simulink model "DPA_6bitDAC_MIXER_INL"  (R2015b)
settings: Solver=FixedStepDiscrete  SolverMode=SingleTasking  StartTime=0.0  StopTime=1/fs*(4*nn+ni)  RelTol=1e-3  AbsTol=1e-6
values from neighbouring files (symbols this model uses):
  AM = 1    [load_6bit_DPA_Mixerpsd_INL.m]
  Fc = 6.5e9    (= 6500000000)    [load_6bit_DPA_Mixerpsd_INL.m]
  fin1 = fs/nn*floor(fin1/fs*nn)    [load_6bit_DPA_Mixerpsd_INL.m]
  fin2 = fs/nn*floor(fin2/fs*nn)    [load_6bit_DPA_Mixerpsd_INL.m]
  fin3 = fs/nn*floor(fin3/fs*nn)    [load_6bit_DPA_Mixerpsd_INL.m]
  fin4 = fs/nn*floor(fin4/fs*nn)    [load_6bit_DPA_Mixerpsd_INL.m]
  fin5 = fs/nn*floor(fin5/fs*nn)    [load_6bit_DPA_Mixerpsd_INL.m]
  fin6 = fs/nn*floor(fin6/fs*nn)    [load_6bit_DPA_Mixerpsd_INL.m]
  fin7 = fs/nn*floor(fin7/fs*nn)    [load_6bit_DPA_Mixerpsd_INL.m]
  fin8 = fs/nn*floor(fin8/fs*nn)    [load_6bit_DPA_Mixerpsd_INL.m]
  fs = Fc*4    (= 26000000000)    [load_6bit_DPA_Mixerpsd_INL.m]
  g1 = (1-2^-32)/8    (= 0.124999999971)    [load_6bit_DPA_Mixerpsd_INL.m]
  NUM = [1,1]    [load_6bit_DPA_Mixerpsd_INL.m]
undefined symbols (not defined in the file or in its folder): RR6bit, RR6bit_ideal
settings Model: ExtModeTrigMode=oneshot  ExtModeArmWhenConnect=off  Creator=john  LastModifiedBy=John_dell_NB2019
settings DataIOCC: LimitDataPoints=off  SaveFormat=Array  SignalLoggingSaveFormat=ModelDataLogs
settings OptimizationCC: BlockReduction=off  BooleanDataType=off
settings DebuggingCC: SaveWithParameterizedLinksMsg=none  UnderspecifiedInitializationDetection=Classic  MergeDetectMultiDrivingBlocksExec=none  SignalResolutionControl=TryResolveAllWithWarning  MultiTaskDSMMsg=warning  MultiTaskCondExecSysMsg=none  StateNameClashWarn=warning
settings HardwareCC: ProdBitPerPointer=32  ProdLargestAtomicFloat=None  ProdIntDivRoundTo=Undefined  ProdEndianess=Unspecified  ProdWordSize=32  ProdHWDeviceType=32-bit Generic  TargetBitPerPointer=64  TargetLongLongMode=on  TargetIntDivRoundTo=Zero  TargetEndianess=LittleEndian  TargetWordSize=64  TargetHWDeviceType=MATLAB Host  ProdEqTarget=off
settings GRTTargetCC: GeneratePreprocessorConditionals=Disable all  CombineOutputUpdateFcns=off  GRTInterface=on
settings ConfigComp: CovModelRefEnable=Off

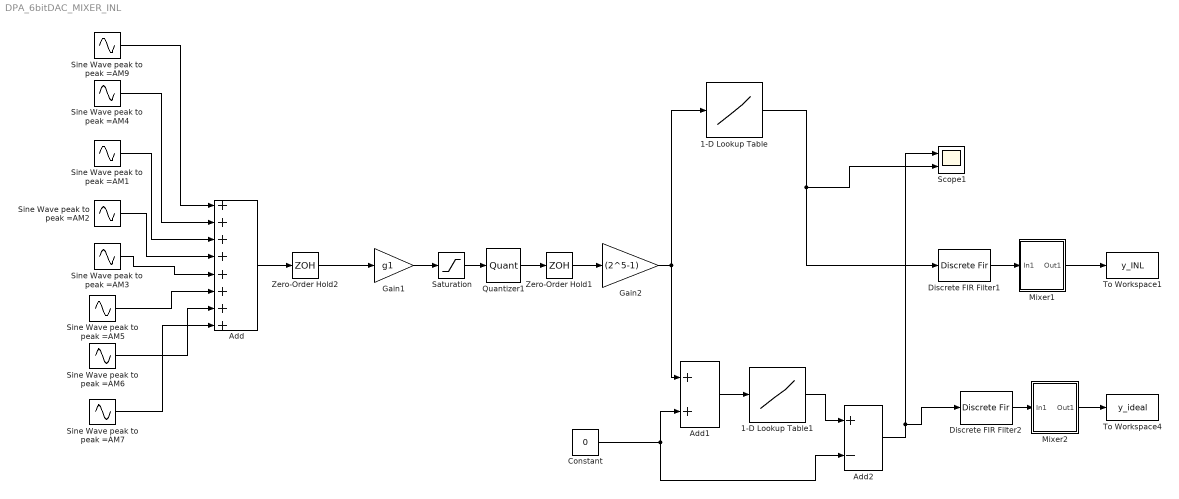
== system DPA_6bitDAC_MIXER_INL ==
  1-D Lookup Table : Lookup_n-D  NumberOfTableDimensions=1  BreakpointsForDimension1=[-31:1:31]  Table=[RR6bit]  InternalRulePriority=Speed  RndMeth=Simplest  InputSameDT=on
  1-D Lookup Table1 : Lookup_n-D  NumberOfTableDimensions=1  BreakpointsForDimension1=[-31:1:31]  Table=[RR6bit_ideal]  InternalRulePriority=Speed  RndMeth=Simplest  InputSameDT=on
  Add : Sum  Inputs=++++++++
  Add1 : Sum
  Add2 : Sum  Inputs=+-
  Constant : Constant  Value=0
  Discrete FIR Filter1 : DiscreteFir  Coefficients=NUM  SampleTime=4/fs
  Discrete FIR Filter2 : DiscreteFir  Coefficients=NUM  SampleTime=4/fs
  Gain1 : Gain  Gain=g1
  Gain2 : Gain  Gain=(2^5-1)
  Mixer1 : Subsystem
  Mixer2 : Subsystem
  Quantizer1 : Quantizer  QuantizationInterval=1/2^(8-1)  LinearizeAsGain=off
  Saturation : Saturate  UpperLimit=1  LowerLimit=-1
  Scope1 : Scope  NumInputPorts=2
  Sine Wave peak to peak =AM1 : Sin  Amplitude=AM  Frequency=2*pi*fin3  SampleTime=8/fs
  Sine Wave peak to peak =AM2 : Sin  Amplitude=AM  Frequency=2*pi*fin4  SampleTime=8/fs
  Sine Wave peak to peak =AM3 : Sin  Amplitude=AM  Frequency=2*pi*fin5  SampleTime=8/fs
  Sine Wave peak to peak =AM4 : Sin  Amplitude=AM  Frequency=2*pi*fin2  SampleTime=8/fs
  Sine Wave peak to peak =AM5 : Sin  Amplitude=AM  Frequency=2*pi*fin6  SampleTime=8/fs
  Sine Wave peak to peak =AM6 : Sin  Amplitude=AM  Frequency=2*pi*fin7  SampleTime=8/fs
  Sine Wave peak to peak =AM7 : Sin  Amplitude=AM  Frequency=2*pi*fin8  SampleTime=8/fs
  Sine Wave peak to peak =AM9 : Sin  Amplitude=AM  Frequency=2*pi*fin1  SampleTime=8/fs
  To Workspace1 : ToWorkspace  VariableName=y_INL  SampleTime=1/fs
  To Workspace4 : ToWorkspace  VariableName=y_ideal  SampleTime=1/fs
  Zero-Order Hold1 : ZeroOrderHold  SampleTime=1/fs
  Zero-Order Hold2 : ZeroOrderHold  SampleTime=8/fs
  wires:
  Sine Wave peak to peak =AM9/1 -> Add/1
  Add/1 -> Zero-Order Hold2/1
  Zero-Order Hold2/1 -> Gain1/1
  Sine Wave peak to peak =AM4/1 -> Add/2
  Sine Wave peak to peak =AM1/1 -> Add/3
  Sine Wave peak to peak =AM2/1 -> Add/4
  Sine Wave peak to peak =AM3/1 -> Add/5
  Sine Wave peak to peak =AM5/1 -> Add/6
  Sine Wave peak to peak =AM6/1 -> Add/7
  Sine Wave peak to peak =AM7/1 -> Add/8
  Saturation/1 -> Quantizer1/1
  Quantizer1/1 -> Zero-Order Hold1/1
  1-D Lookup Table/1 -> Discrete FIR Filter1/1, Scope1/2
  Zero-Order Hold1/1 -> Gain2/1
  Gain2/1 -> Add1/1, 1-D Lookup Table/1
  Gain1/1 -> Saturation/1
  Discrete FIR Filter1/1 -> Mixer1/1(In1)
  Discrete FIR Filter2/1 -> Mixer2/1(In1)
  Mixer1/1(Out1) -> To Workspace1/1
  Mixer2/1(Out1) -> To Workspace4/1
  Add1/1 -> 1-D Lookup Table1/1
  Add2/1 -> Scope1/1, Discrete FIR Filter2/1
  1-D Lookup Table1/1 -> Add2/1
  Constant/1 -> Add2/2, Add1/2

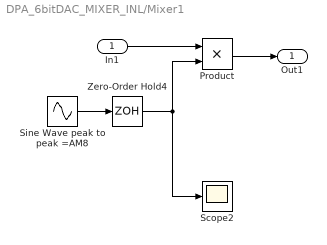
== system DPA_6bitDAC_MIXER_INL/Mixer1 ==
  In1 : Inport
  Product : Product
  Scope2 : Scope
  Sine Wave peak to peak =AM8 : Sin  Amplitude=AM  Frequency=2*pi*Fc  Phase=pi/2  SampleTime=2/fs
  Zero-Order Hold4 : ZeroOrderHold  SampleTime=2/fs
  Out1 : Outport
  wires:
  Sine Wave peak to peak =AM8/1 -> Zero-Order Hold4/1
  In1/1 -> Product/1
  Product/1 -> Out1/1
  Zero-Order Hold4/1 -> Product/2, Scope2/1

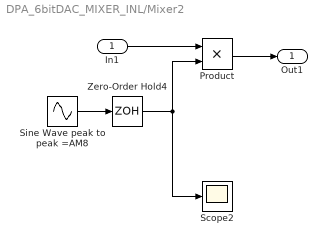
== system DPA_6bitDAC_MIXER_INL/Mixer2 ==
  In1 : Inport
  Product : Product
  Scope2 : Scope
  Sine Wave peak to peak =AM8 : Sin  Amplitude=AM  Frequency=2*pi*Fc  Phase=pi/2  SampleTime=2/fs
  Zero-Order Hold4 : ZeroOrderHold  SampleTime=2/fs
  Out1 : Outport
  wires:
  Sine Wave peak to peak =AM8/1 -> Zero-Order Hold4/1
  In1/1 -> Product/1
  Product/1 -> Out1/1
  Zero-Order Hold4/1 -> Product/2, Scope2/1
